simulink model "ControlledSystem"  (R2020b)
settings: Solver=VariableStepAuto  StartTime=0.0  StopTime=20  RelTol=1e-3
settings Model: Creator=sara6  LastModifiedBy=sara6

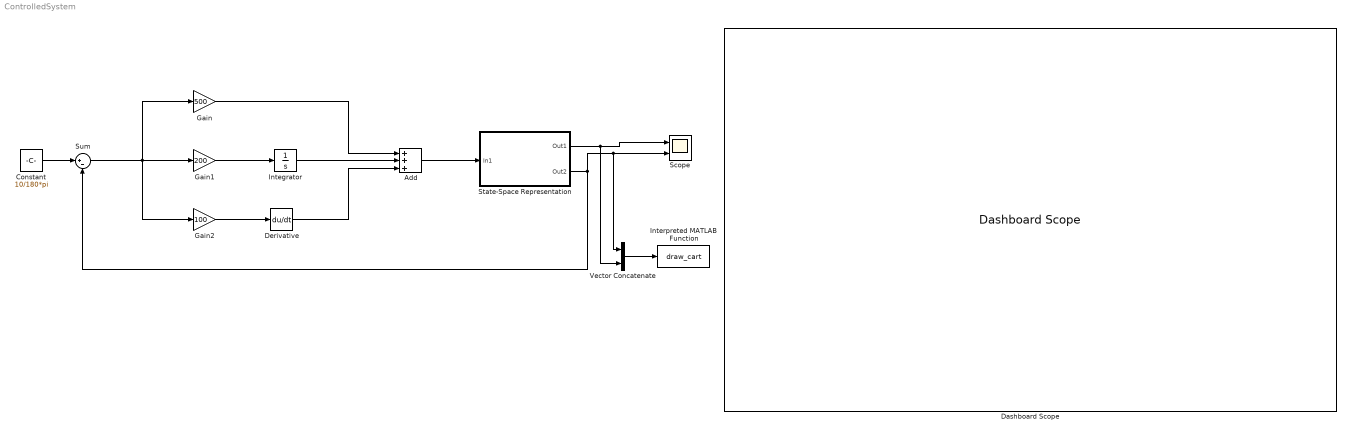
== system ControlledSystem ==
  Add : Sum  Inputs=+++
  Constant : Constant  Value=10/180*pi
  Dashboard Scope : DashboardScope
  Derivative : Derivative
  Gain : Gain  Gain=500
  Gain1 : Gain  Gain=200
  Gain2 : Gain  Gain=100
  Integrator : Integrator
  Interpreted MATLAB Function : MATLABFcn  MATLABFcn=draw_cart  OutputDimensions=0
  Scope : Scope  NumInputPorts=2
  State-Space Representation : Subsystem
  Sum : Sum  Inputs=|+-
  Vector Concatenate : Concatenate
  wires:
  Add/1 -> State-Space Representation/1(In1)
  Gain1/1 -> Integrator/1
  Integrator/1 -> Add/2
  Gain/1 -> Add/1
  Gain2/1 -> Derivative/1
  Derivative/1 -> Add/3
  Sum/1 -> Gain2/1, Gain/1, Gain1/1
  State-Space Representation/1(Out1) -> Vector Concatenate/2, Scope/1
  State-Space Representation/2(Out2) -> Vector Concatenate/1, Scope/2, Sum/2
  Constant/1 -> Sum/1
  Vector Concatenate/1 -> Interpreted MATLAB Function/1

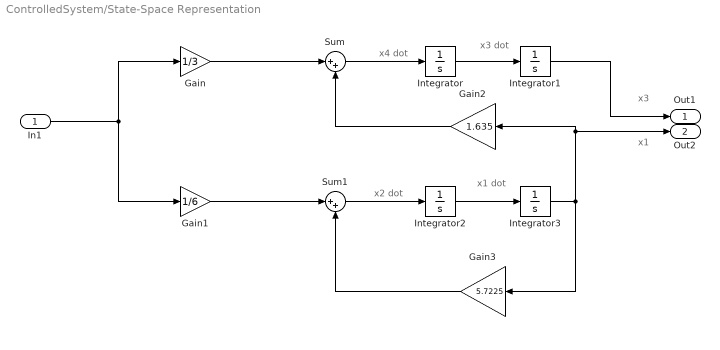
== system ControlledSystem/State-Space Representation ==
  note: x3 dot
  note: x1
  note: x3
  note: x4 dot
  note: x2 dot
  note: x1 dot
  In1 : Inport
  Gain : Gain  Gain=1/3
  Gain1 : Gain  Gain=1/6
  Gain2 : Gain  Gain=1.635
  Gain3 : Gain  Gain=5.7225
  Integrator{,1..3} (4 alike) : Integrator
  Sum : Sum  Inputs=|++
  Sum1 : Sum  Inputs=|++
  Out1 : Outport
  Out2 : Outport  Port=2
  wires:
  Integrator/1 -> Integrator1/1
  Sum1/1 -> Integrator2/1
  Gain2/1 -> Sum/2
  Sum/1 -> Integrator/1
  Integrator3/1 -> Out2/1, Gain2/1, Gain3/1
  Integrator2/1 -> Integrator3/1
  In1/1 -> Gain/1, Gain1/1
  Integrator1/1 -> Out1/1
  Gain/1 -> Sum/1
  Gain1/1 -> Sum1/1
  Gain3/1 -> Sum1/2
